simulink model "LeftCameraAgent"  (Simulink 5.0)
settings: Solver=ode45  StartTime=0.0  StopTime=10.0  RelTol=1e-3
settings Model: LastModifiedBy=suarezjl

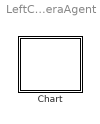
== system LeftCameraAgent ==
  Chart : Stateflow chart

== stateflow chart Chart ==
  state Initial
    \\Sally\LeftCameraAgent\FrameGrabber.Initialize()
    \\Sally\LeftCameraAgent\FrameGrabber.ObtainImage()
    \\Sally\LeftCameraAgent\FrameGrabber.ObtainImage()
    \\Sally\LeftCameraAgent\ColorSegmenter.Initial()
    \\Sally\LeftCameraAgent\ColorSegmenter.LoadColorModel()
  state Segmentation
    \\Sally\LeftCameraAgent\FrameGrabber.ObtainImage()
    \\Sally\LeftCameraAgent\ColorSegmenter.DoSegment()
  (default) -> Initial : Start
  Initial -> Segmentation : Always
  Segmentation -> Segmentation : Always
